simulink model "Quanser_Qube_Plant"  (R2018a)
settings: Solver=ode1  StartTime=0.0  StopTime=inf  FixedStep=0.002  RelTol=1e-3  EnableMultiTasking=on
undefined symbols (not defined in the file or in its folder): HIL, N, qc_get_step_size, w0, wf
libraries: quarc_library x3
settings Model: SimulationMode=external  ExtModeTrigDuration=200000  Creator=MLevis  LastModifiedBy=Joe
settings SolverCC: PositivePriorityOrder=on
settings DataIOCC: LimitDataPoints=on  SaveFormat=Array  SignalLoggingSaveFormat=ModelDataLogs
settings OptimizationCC: BooleanDataType=off  OptimizeBlockIOStorage=off  BufferReuse=off  GlobalBufferReuse=off  ExpressionFolding=off  ExpressionDepthLimit=2147483647  LocalBlockOutputs=off  InitFltsAndDblsToZero=on  LifeSpan=inf  OptimizeDataStoreBuffers=off  BusAssignmentInplaceUpdate=off
settings DebuggingCC: SaveWithParameterizedLinksMsg=none  UnderspecifiedInitializationDetection=Classic  MergeDetectMultiDrivingBlocksExec=none  SignalResolutionControl=TryResolveAllWithWarning  MultiTaskDSMMsg=warning  MultiTaskCondExecSysMsg=none  FcnCallInpInsideContextMsg=warning  StateNameClashWarn=warning  SFUnexpectedBacktrackingDiag=warning  SFNoUnconditionalDefaultTransitionDiag=warning  SFExecutionAtInitializationDiag=none
settings HardwareCC: ProdBitPerPointer=32  ProdBitPerSizeT=32  ProdBitPerPtrDiffT=32  ProdLargestAtomicFloat=None  ProdIntDivRoundTo=Undefined  ProdEndianess=Unspecified  ProdWordSize=32  ProdHWDeviceType=32-bit Generic  TargetHWDeviceType=32-bit Generic
settings ModelReferenceCC: PropagateSignalLabelsOutOfModel=off
settings SFSimCC: SimParseCustomCode=off
settings RTWCC: SystemTargetFile=quarc_win64.tlc  TemplateMakefile=quarc_default_tmf  Description=QUARC Win64 Target
settings CodeAppCC: StateflowObjectComments=on
settings STFCustomTargetCC: TargetPreCompLibLocation=C:\PROGRA~3\QUARC\lib\2018a\win64\release  ConcurrentExecutionCompliant=on  GeneratePreprocessorConditionals=Disable all  SystemTargetFile=quarc_win64.tlc
settings GRTTargetCC: TargetPreCompLibLocation=C:\PROGRA~3\QUARC\lib\2018a\win64\release  TargetLangStandard=C89/C90 (ANSI)  ParMdlRefBuildCompliant=off  CompOptLevelCompliant=off  GeneratePreprocessorConditionals=Disable all  CombineOutputUpdateFcns=off  MatFileLogging=off  CPPClassGenCompliant=off  GRTInterface=on  UseToolchainInfoCompliant=off  ExtMode=on  ExtModeMexFile=quarc_comm
settings ConfigComp: CovMetricSettings=dw  CovHtmlReporting=on  CovSaveCumulativeToWorkspaceVar=on  CovSaveSingleToWorkspaceVar=on  CovExternalEMLEnable=off  CovSFcnEnable=off

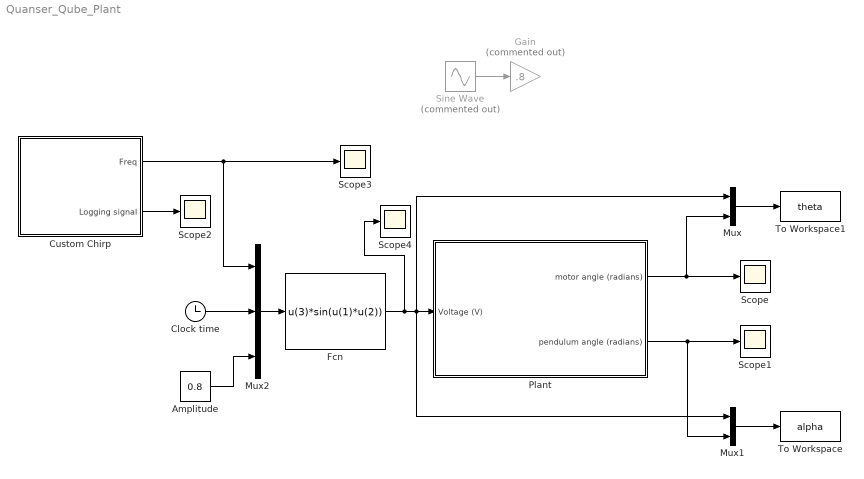
== system Quanser_Qube_Plant ==
  Amplitude : Constant  Value=0.8
  Clock time : Clock
  Custom Chirp : Subsystem
  Fcn : Fcn  Expr=u(3)*sin(u(1)*u(2))
  Gain : Gain  Commented=on  Gain=.8
  Mux : Mux  Inputs=2
  Mux1 : Mux  Inputs=2
  Mux2 : Mux  Inputs=3
  Plant : Subsystem
  Scope{,1..4} (5 alike) : Scope
  Sine Wave : Sin  Commented=on  SampleTime=0
  To Workspace : ToWorkspace  VariableName=alpha  SampleTime=-1
  To Workspace1 : ToWorkspace  VariableName=theta  SampleTime=-1
  wires:
  Sine Wave/1 -> Gain/1
  Plant/1(motor angle (radians)) -> Mux/2, Scope/1
  Fcn/1 -> Scope4/1, Mux/1, Plant/1(Voltage (V)), Mux1/1
  Mux1/1 -> To Workspace/1
  Mux/1 -> To Workspace1/1
  Plant/2(pendulum angle (radians)) -> Mux1/2, Scope1/1
  Custom Chirp/1(Freq) -> Mux2/1, Scope3/1
  Custom Chirp/2(Logging signal) -> Scope2/1
  Mux2/1 -> Fcn/1
  Clock time/1 -> Mux2/2
  Amplitude/1 -> Mux2/3

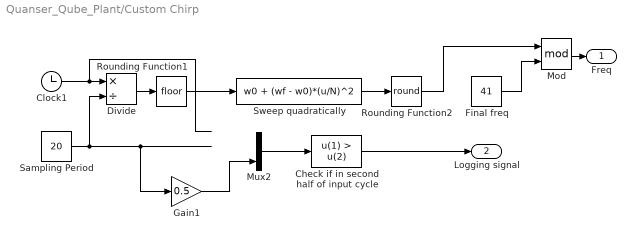
== system Quanser_Qube_Plant/Custom Chirp ==
  Check if in second half of input cycle : Fcn  Expr=u(1) > u(2)
  Clock1 : Clock
  Divide : Product  Inputs=*/
  Final freq : Constant  Value=41
  Gain1 : Gain  Gain=0.5
  Mod : Math  Operator=mod  SaturateOnIntegerOverflow=on
  Mux2 : Mux  Inputs=2
  Rounding Function1 : Rounding
  Rounding Function2 : Rounding  Operator=round
  Sampling Period : Constant  Value=20
  Sweep quadratically : Fcn  Expr=w0 + (wf - w0)*(u/N)^2
  Freq : Outport
  Logging signal : Outport  Port=2
  wires:
  Divide/1 -> Rounding Function1/1
  ? -> Mux2/1
  Sweep quadratically/1 -> Rounding Function2/1
  Clock1/1 -> Divide/1
  Sampling Period/1 -> Gain1/1, Divide/2
  Check if in second half of input cycle/1 -> Logging signal/1
  Mux2/1 -> Check if in second half of input cycle/1
  Rounding Function1/1 -> Sweep quadratically/1
  Gain1/1 -> Mux2/2
  Rounding Function2/1 -> Mod/1
  Final freq/1 -> Mod/2
  Mod/1 -> Freq/1

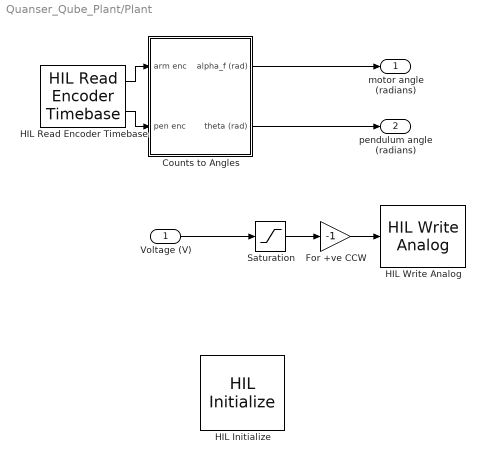
== system Quanser_Qube_Plant/Plant ==
  Voltage (V) : Inport
  Counts to Angles : Subsystem
  For +ve CCW : Gain  Gain=-1
  HIL Initialize : quarc_library/Data Acquisition/Generic/Configuration/HIL Initialize  object_name=HIL-1  board_type=qube_servo2_usb  board_number=0  board_options=""  exclusive=off  active=off  hardware_clocks=[0]  clock_modes=[]  initial_clock_frequencies=[]  set_clock_params_at_start=off  set_clock_params_at_switch_in=off  set_clock_frequencies_at_start=off  set_clock_frequencies_at_switch_in=off  analog_input_channels=[0]  analog_input_configurations=[]  analog_input_maximums=3  analog_input_minimums=-3  set_analog_input_params_at_start=off  set_analog_input_params_at_switch_in=off  analog_output_channels=[0]  analog_output_maximums=15  analog_output_minimums=-15  initial_analog_outputs=[0]  final_analog_outputs=[0]  watchdog_analog_outputs=0  set_analog_output_params_at_start=off  set_analog_output_params_at_switch_in=off  set_analog_outputs_at_start=on  set_analog_outputs_at_switch_in=off  set_analog_outputs_at_terminate=on  set_analog_outputs_at_switch_out=off  set_analog_outputs_on_watchdog=on  digital_input_channels=[]  digital_output_channels=[0]  digital_output_configuration=[]  initial_digital_outputs=[1]  final_digital_outputs=[0]  watchdog_digital_outputs=[0]  set_digital_output_params_at_start=off  set_digital_output_params_at_switch_in=off  set_digital_outputs_at_start=on  set_digital_outputs_at_switch_in=off  set_digital_outputs_at_terminate=on  set_digital_outputs_at_switch_out=off  set_digital_outputs_on_watchdog=on  encoder_channels=[0:1]  quadrature=[4]  encoder_filter_frequency=[]  initial_encoder_counts=[0]  set_encoder_params_at_start=off  set_encoder_params_at_switch_in=off  set_encoder_counts_at_start=on  set_encoder_counts_at_switch_in=off  pwm_channels=[]  pwm_modes=[]  pwm_frequency=[]  pwm_configuration=[]  pwm_alignment=[]  pwm_polarity=[]  pwm_leading_deadband=[]  pwm_trailing_deadband=[]  initial_pwm_outputs=[]  final_pwm_outputs=[]  watchdog_pwm_outputs=[]  set_pwm_params_at_start=off  set_pwm_params_at_switch_in=off  set_pwm_outputs_at_start=off  set_pwm_outputs_at_switch_in=off  set_pwm_outputs_at_terminate=off  set_pwm_outputs_at_switch_out=off  set_pwm_outputs_on_watchdog=off  other_output_channels=[11000:11002]  initial_other_outputs=[0 1 0]  final_other_outputs=[1 0 0]  watchdog_other_outputs=[0 0 1]  set_other_outputs_at_start=on  set_other_outputs_at_switch_in=off  set_other_outputs_at_terminate=on  set_other_outputs_at_switch_out=off  set_other_outputs_on_watchdog=on
  HIL Read Encoder Timebase : quarc_library/Data Acquisition/Generic/Timebases/HIL Read Encoder Timebase  object_name=HIL-1  clock=0  channels=[0:1]  samples_in_buffer=max(ceil(1/qc_get_step_size), 1)  active=on  vector_output=off  data_type_mode=Inherit via back propagation  data_type=double
  HIL Write Analog : quarc_library/Data Acquisition/Generic/Immediate I//O/HIL Write Analog  object_name=HIL-1  channels=0  sample_time=-1  active=off  vector_input=off
  Saturation : Saturate  UpperLimit=10  LowerLimit=-10
  motor angle (radians) : Outport
  pendulum angle (radians) : Outport  Port=2
  wires:
  Counts to Angles/2(theta (rad)) -> pendulum angle (radians)/1
  Counts to Angles/1(alpha_f (rad)) -> motor angle (radians)/1
  HIL Read Encoder Timebase/2 -> Counts to Angles/2(pen enc)
  HIL Read Encoder Timebase/1 -> Counts to Angles/1(arm enc)
  Voltage (V)/1 -> Saturation/1
  Saturation/1 -> For +ve CCW/1
  For +ve CCW/1 -> HIL Write Analog/1

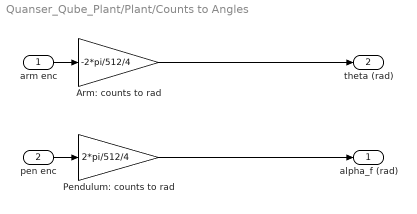
== system Quanser_Qube_Plant/Plant/Counts to Angles ==
  arm enc : Inport
  pen enc : Inport  Port=2
  Arm: counts to rad : Gain  Gain=-2*pi/512/4
  Pendulum: counts to rad : Gain  Gain=2*pi/512/4
  alpha_f (rad) : Outport
  theta (rad) : Outport  Port=2
  wires:
  pen enc/1 -> Pendulum: counts to rad/1
  arm enc/1 -> Arm: counts to rad/1
  Pendulum: counts to rad/1 -> alpha_f (rad)/1
  Arm: counts to rad/1 -> theta (rad)/1
